simulink model "Sposob_4b"  (R2022b)
settings: Solver=ode4  StartTime=0.0  StopTime=10.0  FixedStep=0.1  RelTol=1e-3
values from neighbouring files (symbols this model uses):
  A = [0  1; -0.428571428571  0]    [Sposob2a.mat]    (also in Sposob2b.mat; Sposob4a.mat; Sposob4b.mat)
  B = [0 0]    [Sposob2a.mat]    (also in Sposob2b.mat = [0 0.0714285714286]; Sposob4b.mat = [0 0.0714285714286])
  F = 1    [Sposob1.mat]    (also in Sposob2a.mat; Sposob2b.mat; Sposob3a.mat; Sposob3b.mat)
  x0 = 0.1    [Sposob1.mat]    (also in Sposob2a.mat = [0.1 0]; Sposob2b.mat = [0.1 0]; Sposob3a.mat = [0.1 0]; Sposob3b.mat = [0.1 0])
settings Model: Creator=student  LastModifiedBy=Jakub
settings DebuggingCC: UnconnectedInputMsg=warning  UnconnectedOutputMsg=warning  UnconnectedLineMsg=warning
settings ModelReferenceCC: EnableRefExpFcnMdlSchedulingChecks=on
settings RTWCC: DLArmComputeVersion=19.05

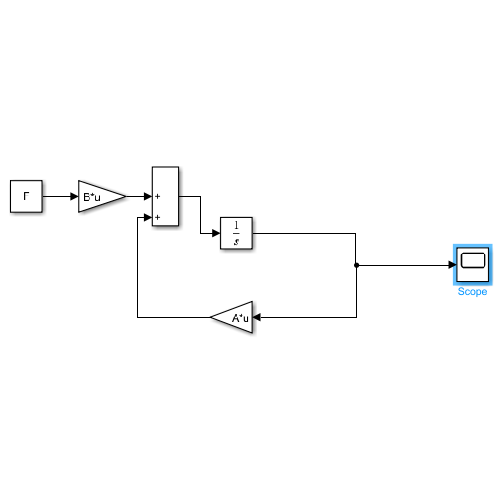
[thumbnail: Simulink's stored preview of the top-level diagram]
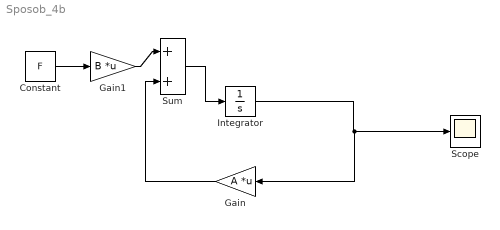
== system Sposob_4b ==
  Constant : Constant  Value=F
  Gain : Gain  Gain=A  Multiplication=Matrix(K*u)
  Gain1 : Gain  Gain=B  Multiplication=Matrix(K*u)
  Integrator : Integrator  InitialCondition=x0
  Scope : Scope
  Sum : Sum  Inputs=|++
  wires:
  Integrator/1 -> Gain/1, Scope/1
  Gain/1 -> Sum/2
  Gain1/1 -> Sum/1
  Constant/1 -> Gain1/1
  Sum/1 -> Integrator/1
